simulink model "Projeto_Final_M21"  (R2021a)
settings: Solver=VariableStepAuto  StartTime=0  StopTime=200  FixedStep=0.1  RelTol=1e-3
model workspace (MAT data in the model file):
  N_P0 = 3
  variavelteste = 0
libraries: spsACVoltageSourceLib x1, autolibsharedmappedengines x1, spsCurrentMeasurementLib x1, spsSeriesRLCBranchLib x1, spspowerguiLib x1
(part 3 of 3)

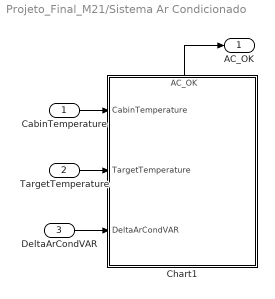
== system Projeto_Final_M21/Sistema Ar Condicionado ==
  CabinTemperature : Inport
  TargetTemperature : Inport  Port=2
  DeltaArCondVAR : Inport  Port=3
  Chart1 : Stateflow chart  TreatAsAtomicUnit=on
      settings: PortSchema="{\"entries\":[{\"content\":{\"sides\":[{\"content\":{\"connectorIds\":[\"In1\",\"In2\",\"In3\"]},\"type\":\"ConnectorPlacement.EquallySpacedRectSide\",\"uuid\":\"3dcc586e-91d0-4cd1-aed7-6dda3adf5149\"},{\"content\":{\"connectorIds\":[],\"side\":\"RIGHT\"},\"type\":\"ConnectorPlacement.EquallySpacedRectSide\",\"uuid\":\"6a827bb4-538e-49ed-9fcc-bcf1675a0976\"},{\"content\":{\"connectorIds\":[\"Out1\"],\"side\":\"TOP\"},\"type\":\"ConnectorPlacement.EquallySpacedRectSide\",\"uuid\":\"8af03e4c-b384-4eb2-b8cc-d6be61dc8da4\"}]},\"type\":\"ConnectorPlacement.EquallySpacedConnector\",\"uuid\":\"bd7ebad6-2738-4989-9528-f935edcb496d\"}],\"packageUris\":[\"http://schema.mathworks.com/mf0/Connector/R2020b\"],\"version\":\"1.0\"}"
  AC_OK : Outport
  wires:
  Chart1/1(AC_OK) -> AC_OK/1
  CabinTemperature/1 -> Chart1/1(CabinTemperature)
  TargetTemperature/1 -> Chart1/2(TargetTemperature)
  DeltaArCondVAR/1 -> Chart1/3(DeltaArCondVAR)

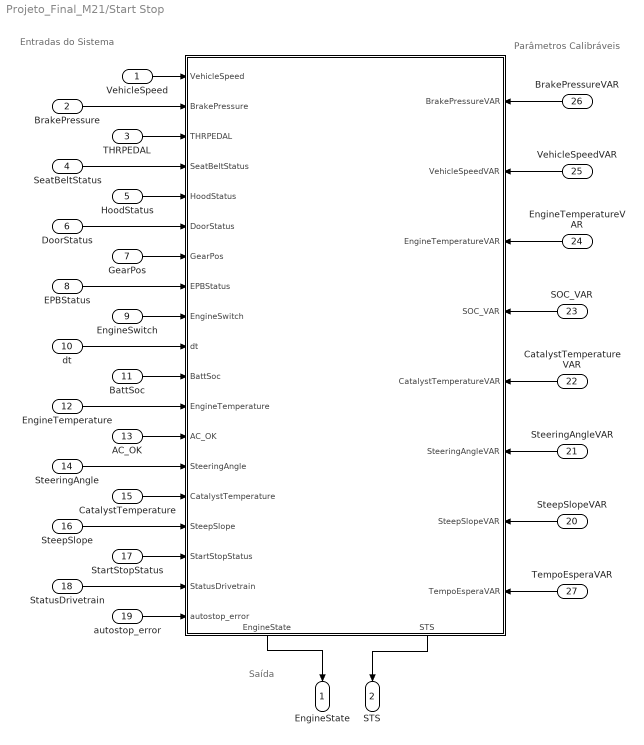
== system Projeto_Final_M21/Start Stop ==
  note: Saída
  note: Entradas do Sistema
  note: Parâmetros Calibráveis
  VehicleSpeed : Inport
  BrakePressure : Inport  Port=2
  THRPEDAL : Inport  Port=3
  SeatBeltStatus : Inport  Port=4
  HoodStatus : Inport  Port=5
  DoorStatus : Inport  Port=6
  GearPos : Inport  Port=7
  EPBStatus : Inport  Port=8
  EngineSwitch : Inport  Port=9
  dt : Inport  Port=10
  BattSoc : Inport  Port=11
  EngineTemperature : Inport  Port=12
  AC_OK : Inport  Port=13
  SteeringAngle : Inport  Port=14
  CatalystTemperature : Inport  Port=15
  SteepSlope : Inport  Port=16
  StartStopStatus : Inport  Port=17
  StatusDrivetrain : Inport  Port=18
  autostop_error : Inport  Port=19
  SteepSlopeVAR : Inport  Port=20
  SteeringAngleVAR : Inport  Port=21
  CatalystTemperatureVAR : Inport  Port=22
  SOC_VAR : Inport  Port=23
  EngineTemperatureVAR : Inport  Port=24
  VehicleSpeedVAR : Inport  Port=25
  BrakePressureVAR : Inport  Port=26
  TempoEsperaVAR : Inport  Port=27
  " " : Stateflow chart  TreatAsAtomicUnit=on
      settings: PortSchema="{\"entries\":[{\"content\":{\"sides\":[{\"content\":{\"connectorIds\":[\"In10\",\"In11\",\"In12\",\"In13\",\"In14\",\"In15\",\"In16\",\"In19\",\"In20\",\"In9\",\"In21\",\"In22\",\"In23\",\"In24\",\"In25\",\"In26\",\"In27\",\"In17\",\"In18\"]},\"type\":\"ConnectorPlacement.EquallySpacedRectSide\",\"uuid\":\"823cfa7e-5a36-4c70-a231-0fae78490b25\"},{\"content\":{\"connectorIds\":[\"In1\",\"In2\",\"In3\",\"In4\",\"In5\",\"In6\",\"In7\",\"In8\"],\"side\":\"RIGHT\"},\"type\":\"ConnectorPlacement.EquallySpacedRectSide\",\"uuid\":\"b0c8ae88-7a9c-4152-8df4-361411c6999f\"},{\"content\":{\"connectorIds\":[],\"side\":\"TOP\"},\"type\":\"ConnectorPlacement.EquallySpacedRectSide\",\"uuid\":\"23b42440-538d-4cea-9d30-9fc9eba2f409\"},{\"content\":{\"connectorIds\":[\"Out1\",\"Out2\"],\"side\":\"BOTTOM\"},\"type\":\"ConnectorPlacement.EquallySpacedRectSide\",\"uuid\":\"b132eeeb-9f39-4852-bf80-9b9b82940eba\"}]},\"type\":\"ConnectorPlacement.EquallySpacedConnector\",\"uuid\":\"9c597531-0edf-4da3-a7a2-f3937f962f4c\"}],\"packageUris\":[\"http://schema.mathworks.com/mf0/Connector/R2020b\"],\"version\":\"1.0\"}"
  EngineState : Outport
  STS : Outport  Port=2
  wires:
  THRPEDAL/1 -> " "/12(THRPEDAL)
  EngineTemperature/1 -> " "/22(EngineTemperature)
  AC_OK/1 -> " "/23(AC_OK)
  BattSoc/1 -> " "/21(BattSoc)
  VehicleSpeed/1 -> " "/10(VehicleSpeed)
  GearPos/1 -> " "/16(GearPos)
  BrakePressure/1 -> " "/11(BrakePressure)
  HoodStatus/1 -> " "/14(HoodStatus)
  DoorStatus/1 -> " "/15(DoorStatus)
  EngineSwitch/1 -> " "/20(EngineSwitch)
  EPBStatus/1 -> " "/19(EPBStatus)
  SeatBeltStatus/1 -> " "/13(SeatBeltStatus)
  SteeringAngle/1 -> " "/24(SteeringAngle)
  CatalystTemperature/1 -> " "/25(CatalystTemperature)
  SteepSlope/1 -> " "/26(SteepSlope)
  StartStopStatus/1 -> " "/27(StartStopStatus)
  " "/1(EngineState) -> EngineState/1
  SteepSlopeVAR/1 -> " "/7(SteepSlopeVAR)
  SteeringAngleVAR/1 -> " "/6(SteeringAngleVAR)
  CatalystTemperatureVAR/1 -> " "/5(CatalystTemperatureVAR)
  SOC_VAR/1 -> " "/4(SOC_VAR)
  EngineTemperatureVAR/1 -> " "/3(EngineTemperatureVAR)
  VehicleSpeedVAR/1 -> " "/2(VehicleSpeedVAR)
  BrakePressureVAR/1 -> " "/1(BrakePressureVAR)
  TempoEsperaVAR/1 -> " "/8(TempoEsperaVAR)
  dt/1 -> " "/9(dt)
  StatusDrivetrain/1 -> " "/17(StatusDrivetrain)
  autostop_error/1 -> " "/18(autostop_error)
  " "/2(STS) -> STS/1

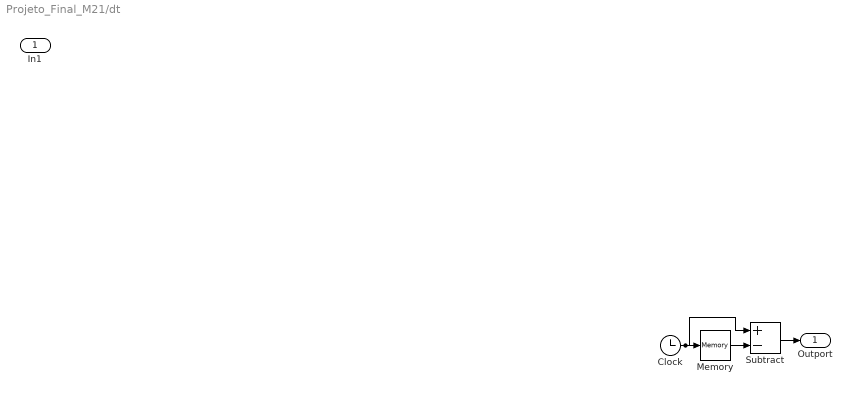
== system Projeto_Final_M21/dt ==
  In1 : Inport
  Clock : Clock
  Memory : Memory
  Subtract : Sum  Inputs=+-
  Outport : Outport
  wires:
  Memory/1 -> Subtract/2
  Clock/1 -> Subtract/1, Memory/1
  Subtract/1 -> Outport/1

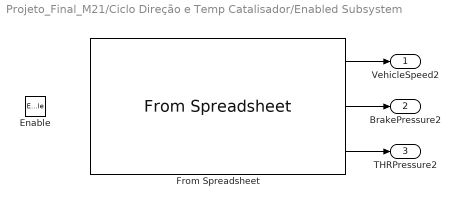
== system Projeto_Final_M21/Ciclo Direção e Temp Catalisador/Enabled Subsystem ==
  Enable : EnablePort
  From Spreadsheet : FromSpreadsheet  FileName=tempo.xlsx  SheetName=tempo  Range=A2:D1512  SampleTime=-1
  VehicleSpeed2 : Outport  InitialOutput=0  VectorParamsAs1DForOutWhenUnconnected=off
  BrakePressure2 : Outport  Port=2  InitialOutput=0  VectorParamsAs1DForOutWhenUnconnected=off
  THRPressure2 : Outport  Port=3
  wires:
  From Spreadsheet/1 -> VehicleSpeed2/1
  From Spreadsheet/2 -> BrakePressure2/1
  From Spreadsheet/3 -> THRPressure2/1

== stateflow chart Projeto_Final_M21/Sistema Ar Condicionado/Chart1 ==
  state AC_Normal
    entry:
    AC_OK = 1;
  state AC_Block
    entry:
    AC_OK = 0;
  (default) -> AC_Normal
  AC_Block -> AC_Normal : [abs(CabinTemperature - TargetTemperature) <= DeltaArCondVAR || abs(TargetTemperature - CabinTemperature) <= DeltaArCondVAR]
  AC_Normal -> AC_Block : [abs(CabinTemperature - TargetTemperature) > DeltaArCondVAR || abs(TargetTemperature - CabinTemperature) > DeltaArCondVAR]
  data: CabinTemperature input; TargetTemperature input double; AC_OK output double; DeltaArCondVAR input

== matlab function Projeto_Final_M21/Ciclo Direção e Temp Catalisador/MATLAB Function ==
  data: Marcha input; Ativar output; EngineSwitch input
function Ativar = AtivarSubSistema(Marcha, EngineSwitch)
%A marcha igual a 3 significa que o carro está no "D" - Modo Drive

if ((Marcha==3) && (EngineSwitch==1))  
    Ativar = 1;
else 
    Ativar = 0;
end

== stateflow chart Projeto_Final_M21/Start Stop/  ==
  state EngineON1
    % Estado de Motor Ligado em Funcionamento Pleno
    entry:
    EngineState = 1;  % Motor ligado
    tempo_espera = 0;  % Reseta o contador ao entrar no estado
    during:
    tempo_espera = 0;  % Sempre zera enquanto está no ON normal
    STS = 0;
  state EngineOFF1
    % Estado de Motor Desligado Inicial
    EngineState = 0;  % Motor desligado
    STS = 0;
  state EPBSecurityActivation
    % Estado de ativação do EPB virtualmente por segurança
    EPBStatus == 1; % Ativa o EPB como medida de segurança Extra
    STS = 0;
  state WaitForAutoStop
    % Estado de Checagem dos Parâmetros do Start/Stop
    entry:
    tempo_espera = 0;  % reseta o timer ao entrar
    during:
    tempo_espera = tempo_espera + dt;
    STS = 1;
  state WaitToTurnOnDef
    % Estado intermediário entre Motor ligado em pleno funcionamento
    EngineState = 1;  % Motor ligado
    STS = 0;
  state EPBSecurityDeactivation
    % Estado de desativação do EPB virtual
    EPBStatus == 0;
    STS = 0;
  state AutoStop1
    % Estado de atuação do Start/Stop
    EngineState = 0;  % Motor desligado temporariamente
    STS = 1;
  EngineON1 -> WaitForAutoStop [order 2] : [((GearPos == 3) || (GearPos == 2)) && ...
      | (AC_OK == 1) && (StartStopStatus ==1) && (EPBStatus == 0) && ...
      | (SeatBeltStatus == 1) && (HoodStatus == 1) && (DoorStatus == 1) && ...
      | (StatusDrivetrain == 1) && (autostop_error == 0) && ...
      | (BrakePressure > BrakePressureVAR) && ...
      | (EngineTemperature > EngineTemperatureVAR) && ...
      | (BattSoc >= SOC_VAR) && (VehicleSpeed==VehicleSpeedVAR) && ...
      | (CatalystTemperature > CatalystTemperatureVAR) && ...
      | (SteeringAngle < SteeringAngleVAR) && (-SteeringAngleVAR < SteeringAngle) && ...
      | (SteepSlope < SteepSlopeVAR)]
  EngineOFF1 -> EngineON1 : [EngineSwitch == 1]
  EngineON1 -> EPBSecurityActivation [order 3] : [(DoorStatus == 0) && (SeatBeltStatus == 0) && ...
      | (BrakePressure == 0) && (GearPos ~= 1)]
  EngineON1 -> EngineOFF1 [order 1] : [(EngineSwitch == 0) && (GearPos == 1)]
  WaitToTurnOnDef -> EngineON1 [order 1] : [hasChanged(VehicleSpeed)]
  (default) -> EngineOFF1
  WaitToTurnOnDef -> EngineOFF1 [order 3] : [(EngineSwitch == 0) && (GearPos == 1)]
  WaitToTurnOnDef -> EPBSecurityActivation [order 2] : [(DoorStatus == 0) && (SeatBeltStatus == 0) && ...
      | (BrakePressure == 0) && (GearPos ~= 1) && ...
      | (EPBStatus == 0) && VehicleSpeed == 0]
  EPBSecurityActivation -> EPBSecurityDeactivation : [(BrakePressure > 0) || ...
      | (THRPEDAL > 0) || ...
      | (EPBStatus == 0)]
  EPBSecurityDeactivation -> WaitToTurnOnDef
  WaitForAutoStop -> WaitToTurnOnDef [order 2] : [(autostop_error == 1)]
  WaitForAutoStop -> AutoStop1 [order 1] : [(tempo_espera >= TempoEsperaVAR) && ...
      | (autostop_error == 0)]
  AutoStop1 -> WaitToTurnOnDef : [(BrakePressure <= BrakePressureVAR*0.5) || (AC_OK == 0) || ...
      | (BattSoc < SOC_VAR) || (EPBStatus == 1) || ...
      | (GearPos == 4) || (GearPos == 1) || ...
      | (DoorStatus == 0) || (SeatBeltStatus == 0) || ...
      | hasChanged(SteeringAngle) || (autostop_error == 1)]
  data: BrakePressureVAR input; VehicleSpeedVAR input; EngineTemperatureVAR input; SOC_VAR input; CatalystTemperatureVAR input; SteeringAngleVAR input; SteepSlopeVAR input; TempoEsperaVAR input; dt input; VehicleSpeed input; BrakePressure input; THRPEDAL input; SeatBeltStatus input; HoodStatus input; DoorStatus input; GearPos input; StatusDrivetrain input; autostop_error input; EPBStatus input; EngineSwitch input double; tempo_espera local double =0; BattSoc input; EngineTemperature input; AC_OK input; tempoespera local double =0; SteeringAngle input; CatalystTemperature input; SteepSlope input; StartStopStatus input; EngineState output; STS output

== matlab function Projeto_Final_M21/Ciclo Direção e Temp Catalisador/Inverte Sinal do torque aceleraçãoXdesaceleração ==
  data: EngTrq input; EngTrqSaida output; derivada input
function EngTrqSaida = SinalDoTorque(EngTrq,derivada)

%derivada positiva sinal positivo, derivada negativa sinal de saida
%negativo

if (derivada>0)  
    EngTrqSaida = EngTrq;
else 
    EngTrqSaida = -EngTrq;
end

== matlab function Projeto_Final_M21/Condições para o Dashboard ==
  data: SteeringAngle input; SteeringAngleVAR input; Dash_Volante output; Dash_TempMotor output; EngineTemperature input; EngineTemperatureVAR input; BattSoc input; SOC_VAR input; Dash_Bat output; SteepSlope input; SteepSlopeVAR input; Dash_SteepSlope output; InputFalha input; MsgFalha output; STS input; Dash_Running output; CatalystTempVar input; CatalystTemp input; Dash_Catalyst output; EPBStatus input; DoorStatus input; SeatBeltStatus input; BrakePressure input; GearPos input; Dash_EPB output; VehicleSpeed input
function [Dash_Volante,Dash_TempMotor,Dash_Bat,Dash_SteepSlope,MsgFalha,Dash_Running,Dash_Catalyst,Dash_EPB]= ...
          Dashboard(SteeringAngle,SteeringAngleVAR,EngineTemperature, ...
          EngineTemperatureVAR,BattSoc,SOC_VAR,SteepSlope,SteepSlopeVAR, InputFalha, STS,CatalystTempVar,CatalystTemp,EPBStatus,...
          DoorStatus, SeatBeltStatus,BrakePressure,GearPos,VehicleSpeed)
%#codegen

if ((SteeringAngle < SteeringAngleVAR) && (-SteeringAngleVAR < SteeringAngle))
    Dash_Volante = 1;
else
    Dash_Volante = 0;
end 

if (EngineTemperature > EngineTemperatureVAR)
    Dash_TempMotor = 1;
else
    Dash_TempMotor = 0;
end 

if BattSoc >= SOC_VAR
    Dash_Bat = 1;
else 
    Dash_Bat = 0;
end

if SteepSlope < SteepSlopeVAR
    Dash_SteepSlope = 1;
else
    Dash_SteepSlope = 0;
end

%
if InputFalha == 1
    MsgFalha = 1;
else
    MsgFalha = 0;
end

if InputFalha == 0 && STS == 0 
    Dash_Running = 0;  
elseif InputFalha == 0 && STS == 1 
    Dash_Running = 1;  
elseif InputFalha == 1
    Dash_Running = 2;
else
    Dash_Running = 2;
end


%Condição para XX

if CatalystTemp < CatalystTempVar
    Dash_Catalyst = 0;
else
    Dash_Catalyst = 1;
end

if ((DoorStatus == 0) && (SeatBeltStatus == 0) && ...
    (BrakePressure == 0) && (GearPos ~= 1) && ...
    (EPBStatus == 0) && VehicleSpeed == 0)
    Dash_EPB = 2;
elseif EPBStatus == 0
    Dash_EPB = 0;
else 
    Dash_EPB = 1;
end
